simulink model "sistema_motore"  (R2020b)
settings: Solver=VariableStepAuto  StartTime=0.0  StopTime=20  RelTol=1e-3
values from neighbouring files (symbols this model uses):
  A = [0 1 0 0; -k1/m -b1/m 0 0; 0 0 0 1; 0 0 -k2/M -b2/M]    [motore_sistema.m]
  B = [0 0 0 0; -(k1*r3)/m -(b1*r3)/m cos(gamma) 0;0 0 0 0; (k2*r2)/M (b2*r2)/M cos(beta) 0]    [motore_sistema.m]
  C = [+r3*k1 +r3*b1 -r2*k2 -r2*b2; 1 0 0 0; 0 0 1 0]    [motore_sistema.m]
  D = [+(r2^2)*k2+(r3^2)*k1 +(r2^2)*b2+(r3^2)*b1 0 J; 0 0 0 0; 0 0 0 0]    [motore_sistema.m]
  g = 9.81    [motore_sistema.m]
  r1 = 0.05    [motore_sistema.m]
  rm = 0.005    [motore_sistema.m]
  xc = [0 0 0 0]'    [motore_sistema.m]
  xm = [0 0 0]    [motore_sistema.m]
settings Model: Creator=Lenovo  LastModifiedBy=Lenovo

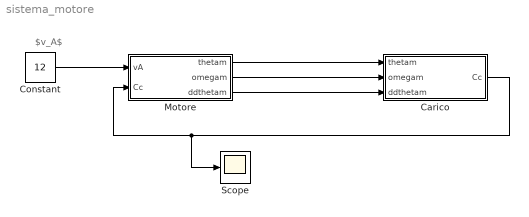
== system sistema_motore ==
  note: $v_A$
  Carico : Subsystem
  Constant : Constant  Value=12
  Motore : Subsystem
  Scope : Scope
  wires:
  Constant/1 -> Motore/1(vA)
  Carico/1(Cc) -> Scope/1, Motore/2(Cc)
  Motore/1(thetam) -> Carico/1(thetam)
  Motore/2(omegam) -> Carico/2(omegam)
  Motore/3(ddthetam) -> Carico/3(ddthetam)

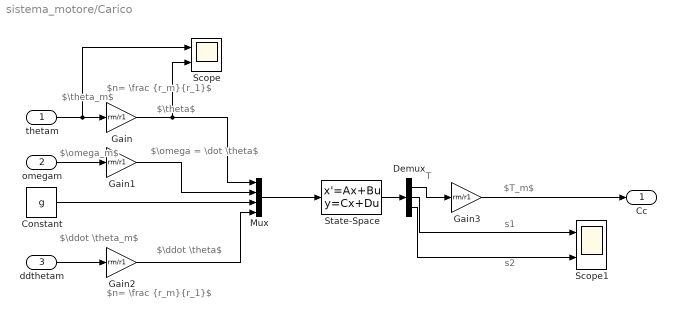
== system sistema_motore/Carico ==
  note: s2
  note: s1
  note: $T_m$
  note: T
  note: $\theta$
  note: $\omega = \dot \theta$
  note: $\ddot \theta$
  note: $\ddot \theta_m$
  note: $\omega_m$
  note: $n= \frac {r_m}{r_1}$
  note: $\theta_m$
  note: $n= \frac {r_m}{r_1}$
  thetam : Inport
  omegam : Inport  Port=2
  ddthetam : Inport  Port=3
  Constant : Constant  Value=g
  Demux : Demux  Outputs=3
  Gain{,1..3} (4 alike) : Gain  Gain=rm/r1
  Mux : Mux
  Scope : Scope  NumInputPorts=2
  Scope1 : Scope  NumInputPorts=2
  State-Space : StateSpace  A=A  B=B  C=C  D=D  InitialCondition=xc
  Cc : Outport
  wires:
  Constant/1 -> Mux/3
  thetam/1 -> Scope/1, Gain/1
  omegam/1 -> Gain1/1
  ddthetam/1 -> Gain2/1
  Gain/1 -> Scope/2, Mux/1
  Gain1/1 -> Mux/2
  Mux/1 -> State-Space/1
  Gain2/1 -> Mux/4
  Gain3/1 -> Cc/1
  State-Space/1 -> Demux/1
  Demux/1 -> Gain3/1
  Demux/2 -> Scope1/1
  Demux/3 -> Scope1/2

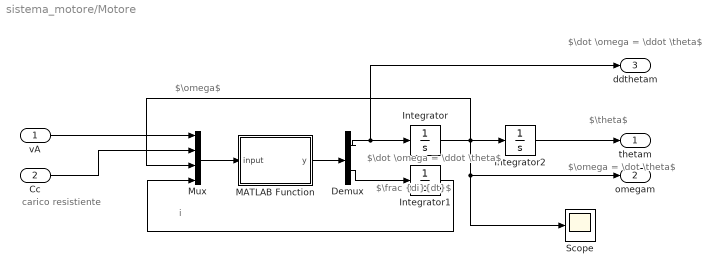
== system sistema_motore/Motore ==
  note: $\omega$
  note: i
  note: $\frac {di}{dt}$
  note: $\dot \omega = \ddot \theta$
  note: $\omega = \dot \theta$
  note: $\theta$
  note: carico resistiente
  note: $\dot \omega = \ddot \theta$
  vA : Inport
  Cc : Inport  Port=2
  Demux : Demux  Outputs=2
  Integrator : Integrator  InitialCondition=xm(2)
  Integrator1 : Integrator  InitialCondition=xm(3)
  Integrator2 : Integrator  InitialCondition=xm(1)
  MATLAB Function : MATLAB Function  TreatAsAtomicUnit=on
  Mux : Mux
  Scope : Scope
  thetam : Outport
  omegam : Outport  Port=2
  ddthetam : Outport  Port=3
  wires:
  Mux/1 -> MATLAB Function/1(input)
  vA/1 -> Mux/1
  Cc/1 -> Mux/2
  MATLAB Function/1(y) -> Demux/1
  Demux/1 -> ddthetam/1, Integrator/1
  Demux/2 -> Integrator1/1
  Integrator1/1 -> Mux/4
  Integrator/1 -> Scope/1, omegam/1, Mux/3, Integrator2/1
  Integrator2/1 -> thetam/1

== matlab function sistema_motore/Motore/MATLAB Function ==
  data: input input; y output
function y = fcn(input)

Ra=0.4;
L=0.2*1e-3;
bm=0.0072;
kc=0.02;
kv=0.02;
Jm=0.002;
y = [0 0]'; 

vA = input (1);
Cc = input (2);
omega = input (3);
i = input (4);

%%y1=domega, y2=di
y(1) = -(bm/Jm)*omega+(kc/Jm)*i-(Cc/Jm);
y(2) = -(Ra/L)*i+(vA/L)-(kv/L)*omega;
